simulink model "Class9_8"  (R2020a)
settings: Solver=VariableStepAuto  StartTime=0.0  StopTime=10.0  RelTol=1e-3
settings Model: Creator=fould  LastModifiedBy=fould

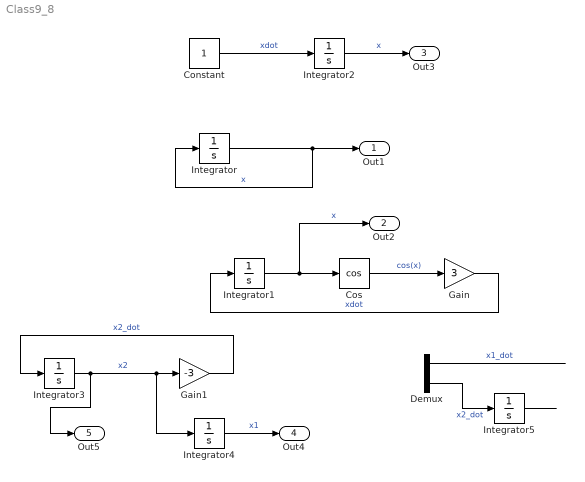
== system Class9_8 ==
  Constant : Constant
  Cos : Trigonometry  Operator=cos
  Demux : Demux  Outputs=2
  Gain : Gain  Gain=3
  Gain1 : Gain  Gain=-3
  Integrator : Integrator  InitialCondition=1
  Integrator1 : Integrator  InitialCondition=1
  Integrator2 : Integrator
  Integrator3 : Integrator  InitialCondition=-2
  Integrator4 : Integrator  InitialCondition=4
  Integrator5 : Integrator
  Out1 : Outport  SignalName=x1
  Out2 : Outport  Port=2  SignalName=x2
  Out3 : Outport  Port=3  SignalName=x3
  Out4 : Outport  Port=4  SignalName=x11
  Out5 : Outport  Port=5  SignalName=x22
  wires:
  Integrator/1 -> Integrator/1, Out1/1  "x"
  Cos/1 -> Gain/1  "cos(x)"
  Integrator1/1 -> Out2/1, Cos/1  "x"
  Gain/1 -> Integrator1/1  "xdot"
  Constant/1 -> Integrator2/1  "xdot"
  Integrator2/1 -> Out3/1  "x"
  Gain1/1 -> Integrator3/1  "x2_dot"
  Integrator3/1 -> Out5/1, Integrator4/1, Gain1/1  "x2"
  ? -> Demux/1  "[x1_dot x2_dot]"
  Demux/1 -> ?  "x1_dot"
  Demux/2 -> Integrator5/1  "x2_dot"
  Integrator5/1 -> ?
  Integrator4/1 -> Out4/1  "x1"
